simulink model "sf_combined_state_actions"  (R2017b)
settings: Solver=FixedStepDiscrete  StartTime=0.0  StopTime=5.0  RelTol=1e-3  EnableMultiTasking=on
settings Model: Creator=The MathWorks, Inc.  LastModifiedBy=The MathWorks, Inc.
settings DataIOCC: LimitDataPoints=on  SaveFormat=Array
settings OptimizationCC: ExpressionDepthLimit=2147483647  LifeSpan=inf
settings DebuggingCC: UnderspecifiedInitializationDetection=Classic  MergeDetectMultiDrivingBlocksExec=none  FcnCallInpInsideContextMsg=warning  StateNameClashWarn=warning  SFUnexpectedBacktrackingDiag=warning  SFNoUnconditionalDefaultTransitionDiag=warning  SFExecutionAtInitializationDiag=none
settings HardwareCC: ProdBitPerPointer=32  ProdBitPerSizeT=32  ProdBitPerPtrDiffT=32  ProdLargestAtomicFloat=None  ProdIntDivRoundTo=Undefined  ProdEndianess=Unspecified  ProdWordSize=32  ProdHWDeviceType=32-bit Generic
settings ModelReferenceCC: PropagateSignalLabelsOutOfModel=off
settings SFSimCC: SimParseCustomCode=off
settings CodeAppCC: StateflowObjectComments=on
settings GRTTargetCC: TargetLangStandard=C89/C90 (ANSI)  GeneratePreprocessorConditionals=Disable all  CombineOutputUpdateFcns=off  GRTInterface=on
settings ConfigComp: CovMetricSettings=dw  CovHtmlReporting=on  CovSaveCumulativeToWorkspaceVar=on  CovSaveSingleToWorkspaceVar=on  CovExternalEMLEnable=off  CovSFcnEnable=off

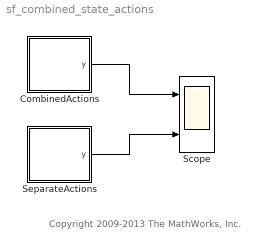
== system sf_combined_state_actions ==
  note: Copyright 2009-2013 The MathWorks, Inc.
  CombinedActions : Stateflow chart  TreatAsAtomicUnit=on
  Scope : Scope  NumInputPorts=2
  SeparateActions : Stateflow chart  TreatAsAtomicUnit=on
  wires:
  CombinedActions/1(y) -> Scope/1
  SeparateActions/1(y) -> Scope/2

== stateflow chart sf_combined_state_actions/CombinedActions ==
  state A
    en: y=0;
    en, du: y++;
  state B
  A -> B : after(5,tick)
  (default) -> A
  data: y output double

== stateflow chart sf_combined_state_actions/SeparateActions ==
  state A
    en: y=0;
    en: y++;
    du: y++;
  state B
  A -> B : after(5,tick)
  (default) -> A
  data: y output double
